simulink model "LVConstant"  (R2020b)
settings: Solver=VariableStepAuto  StartTime=0.0  StopTime=10.0  RelTol=1e-3
values from neighbouring files (symbols this model uses):
  U2 = ui(2)    [Curva_linealidad.m]    (also in FindEquations.m; Horario.m = 0; Linealizar.m = ui(2) + deltau; Untitled.m = 20)
settings Model: Creator=sofia  LastModifiedBy=sofia
settings DataIOCC: SaveOutput=off  SignalLogging=off  DSMLogging=off  SaveTime=off  ReturnWorkspaceOutputs=off

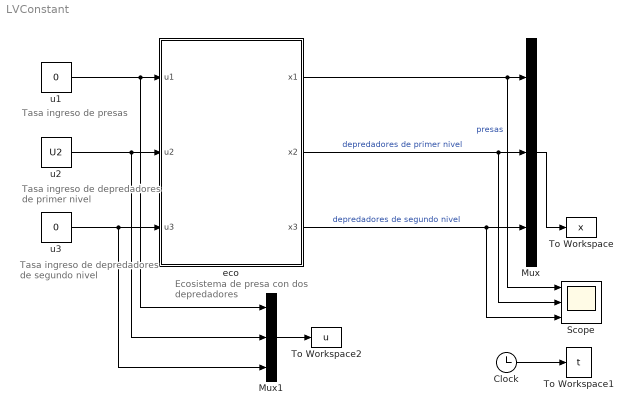
== system LVConstant ==
  note: Tasa ingreso de
      |  depredadores
      | de primer nivel
  note: Ecosistema de presa con
      | dos depredadores
  note: Tasa ingreso de
      |  depredadores
      | de segundo nivel
  note: Tasa ingreso de
      | presas
  Clock : Clock
  Mux : Mux  Inputs=3
  Mux1 : Mux  Inputs=3
  Scope : Scope  NumInputPorts=3
  To Workspace : ToWorkspace  VariableName=x  SampleTime=-1
  To Workspace1 : ToWorkspace  VariableName=t  SampleTime=-1
  To Workspace2 : ToWorkspace  VariableName=u  SampleTime=-1
  eco : Subsystem  mask{ci=[704.569      130.4203      13.04203], ri=[2.84         1.5        0.62], K=8640, ic=[0.02           0        0.03], pc=[0.22           0         0.1]}
      mask prompts: ci "Poblaciones iniciales [x10 x20 x30]"; ri "Tasas de crecimiento intrínseco  [r1 r2 r3]"; K "Capacidad de carga de las presas (K)"; ic "Constantes de interacción [a b c]"; pc "Constantes de proporcionalidad para la capacidad de carga [alpha beta chi]"
      mask init:
      | r1 = ri(1);
      | r2 = ri(2);
      | r3 = ri(3);
      | 
      | 
      | a = ic(1);
      | b = ic(2);
      | c = ic(3);
      | 
      | alpha = pc(1);
      | beta = pc(2);
      | chi = pc(3);
      | 
      | x10 = ci(1);
      | x20 = ci(2);
      | x30 = ci(3);
  u1 : Constant  Value=0
  u2 : Constant  Value=U2
  u3 : Constant  Value=0
  wires:
  u1/1 -> Mux1/1, eco/1(u1)
  Mux1/1 -> To Workspace2/1
  Mux/1 -> To Workspace/1
  Clock/1 -> To Workspace1/1
  eco/3("x3 ") -> Scope/3, Mux/3  "depredadores de segundo nivel"
  eco/2("x2 ") -> Scope/2, Mux/2  "depredadores de primer nivel"
  u3/1 -> Mux1/3, eco/3(u3)
  eco/1("x1 ") -> Scope/1, Mux/1  "presas"
  u2/1 -> Mux1/2, eco/2(u2)

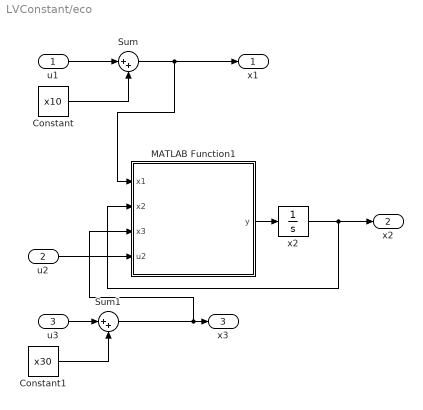
== system LVConstant/eco ==
  u1 : Inport
  u2 : Inport  Port=2
  u3 : Inport  Port=3
  Constant : Constant  Value=x10
  Constant1 : Constant  Value=x30
  MATLAB Function1 : MATLAB Function  TreatAsAtomicUnit=on
  Sum : Sum  Inputs=|++
  Sum1 : Sum  Inputs=|++
  x2 : Integrator  InitialCondition=x20  LimitOutput=on  LowerSaturationLimit=0
  "x1 " : Outport
  "x2 " : Outport  Port=2
  "x3 " : Outport  Port=3
  wires:
  MATLAB Function1/1(y) -> x2/1
  Sum1/1 -> "x3 "/1, MATLAB Function1/3(x3)
  x2/1 -> "x2 "/1, MATLAB Function1/2(x2)
  u2/1 -> MATLAB Function1/4(u2)
  u3/1 -> Sum1/1
  u1/1 -> Sum/1
  Constant/1 -> Sum/2
  Constant1/1 -> Sum1/2
  Sum/1 -> MATLAB Function1/1(x1), "x1 "/1

== matlab function LVConstant/eco/MATLAB Function1 ==
  data: r2 parameter; alpha parameter; c parameter; y output; x1 input; x2 input; x3 input; u2 input
function y = fcn(r2,alpha,c,x1,x2,x3,u2)
    term=0;
    if alpha ~=0
        term = (x2/(alpha*x1));
        y = r2*x2*(1-term)-c*x2*x3+u2;
    else
        y = 0;
    end
end
